simulink model "Simu2VITA"  (R2019b)
settings: Solver=VariableStepAuto  StartTime=0.0  StopTime=10.0  RelTol=1e-3
values from neighbouring files (symbols this model uses):
  actuators_tconst = ones(qty_actuators, 1)*0.1754    [vehicle_parameters_vita1_simu2vita.m]
  Dlf = -[X_u;         Y_v;         Z_w;         K_p;         M_q;         N_r]    [vehicle_parameters_vita1_simu2vita.m]
  Dqf = -[X_u_u;         Y_v_v;         Z_w_w;         K_p_p;         M_q_q;         N_r_r]    [vehicle_parameters_vita1_simu2vita.m]
  I_b = diag([I_x; I_y; I_z])    [vehicle_parameters_vita1_simu2vita.m]
  init_vehicle_linear_vel = [0 0 0]'    [init_params.m]
  init_vehicle_position = [0 0 0]'    [init_params.m]
  m = 25    [vehicle_parameters_vita1_simu2vita.m]
  Ma = -diag([X_u_dot; Y_v_dot; Z_w_dot; K_p_dot; M_q_dot; N_r_dot])    [vehicle_parameters_vita1_simu2vita.m]
  qty_actuators = 8    [vehicle_parameters_vita1_simu2vita.m]
  r_b = [0; 0; -0.08]    [vehicle_parameters_vita1_simu2vita.m]
  r_g = [0; 0; 0.02]    [vehicle_parameters_vita1_simu2vita.m]
  rho = 1028    [vehicle_parameters_vita1_simu2vita.m]
  thrust_inferior = ones(qty_actuators, 1)*(-39.91)    [vehicle_parameters_vita1_simu2vita.m]
  thrust_sup = ones(qty_actuators, 1)*51.48    [vehicle_parameters_vita1_simu2vita.m]
  vol = 0.02432    [vehicle_parameters_vita1_simu2vita.m]
undefined symbols (not defined in the file or in its folder): thruster_allocation_matrix
libraries: sharedutil x3, aerolibutil x3
settings Model: Creator=spades  LastModifiedBy=spades

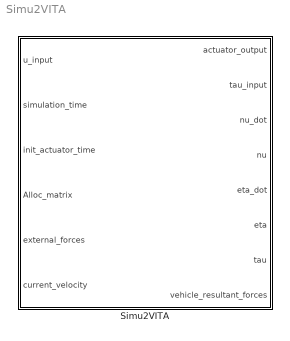
== system Simu2VITA ==
  Simu2VITA : Subsystem  mask{m_qty_actuators=qty_actuators, m_init_actuators_state=0, m_logic_op_use_custom_actuators_init_states=off, m_internal_init_actuators_time=0, m_logic_op_use_external_actuators_init_time=off, m_logic_op_use_external_time=off, m_thrust_sup=thrust_sup, m_thrust_inf=thrust_inferior, m_logic_op_thrust_saturation=on, m_actuators_tconst_vec=actuators_tconst, m_allocation_matrix=thruster_allocation_matrix, m_logic_op_external_alloc_mat=off, m_m=m, m_vol=vol, m_r_g=r_g, m_I_b=I_b, m_loigc_op_use_external_forces=off, m_Ma=Ma, m_Dlf_vec=Dlf, m_Dqf_vec=Dqf, m_current_velocity=[0 0 0]', m_loigc_op_use_external_current_velocity=off, m_g=9.81, m_rho=rho, m_r_b=r_b, m_eta_0=[init_vehicle_position' init_vehicle_orientation']', m_nu_0=[init_vehicle_linear_vel' init_vehicle_angular_vel']'}
      mask prompts: m_qty_actuators "Number of actuators on vehicle"; m_init_actuators_state "Actuators initial state values"; m_logic_op_use_custom_actuators_init_states "use custom initial state for actuators to start"; m_internal_init_actuators_time "Actuators initial time values"; m_logic_op_use_external_actuators_init_time "use external initial time for actuators to start"; m_logic_op_use_external_time "use external clock reference"; m_thrust_sup "Thrust upper saturation limits"; m_thrust_inf "Thrust lower saturation limits"; m_logic_op_thrust_saturation "use thrust saturation"; m_actuators_tconst_vec "Time Constant values"; m_allocation_matrix "Allocation Matrix"; m_logic_op_external_alloc_mat "use external allocation matrix"; m_m "Vehicle Total Mass"; m_vol "Vehicle Total Volume"; m_r_g "Vehicle center of gravity w.r.t. vehicle control point"; m_I_b "Inertia Matrix"; m_loigc_op_use_external_forces "enable external forces and moments"; m_Ma "Addded Mass Matrix"; m_Dlf_vec "Drag Linear Factor"; m_Dqf_vec "Drag Non Linear Factor"; m_current_velocity "Fluid current velocity"; m_loigc_op_use_external_current_velocity "use external fluid current velocity"; m_g "Gravity Constant"; m_rho "Fluid Constant"; m_r_b "Vehicle center of bouyance w.r.t. vehicle body frame"; m_eta_0 "Initial pose of the vehicle -- [pos quat]'"; m_nu_0 "Initial velocity and gyros of the vehicle -- [u v w p q r]'"
      mask init:
      | assert((numel(m_qty_actuators) == 1 && m_qty_actuators >= 0), 'The number of actuators must be a non-negative   scalar.');
      | 
      | if(m_qty_actuators == 0)
      |    
      |     m_logic_op_external_alloc_mat = false;
      |     m_allocation_matrix = zeros(6,1);
      |     m_init_actuators_state = 0;
      |     m_internal_init_actuators_time = 0;
      |     m_actuators_tconst_vec = 1;
      |     m_thrust_sup = 0;
      |     m_thrust_inf = 0;
      |     m_logic_op_thrust_saturation = false;
      |     
      | else
      |     
      |     if(~m_logic_op_use_custom_actuators_init_states)
      |         m_init_actuators_state = zeros(m_qty_actuators,1);
      |     end
      |     
      |     if(~m_logic_op_use_external_actuators_init_time)
      |         
      |         if(m_internal_init_actuators_time == 0)
      |             m_internal_init_actuators_time = zeros(m_qty_actuators,1);
      |         end
      |         
      |     end
      |     
      |     if(m_logic_op_thrust_saturation)
      |         assert(isequal(size(m_thrust_sup), [m_qty_actuators 1]));
      |         assert(isequal(size(m_thrust_inf), [m_qty_actuators 1]));
      |     end
      |     
      |     assert(isequal(size(m_init_actuators_state), [m_qty_actuators 1]), ...
      |         'Initial actuator state vector must be a column vector and agree with the number of actuators specified.');
      |     
      |     assert(isequal(size(m_internal_init_actuators_time), [m_qty_actuators 1]), ...
      |         'Initial actuator time vector must be a column vector and agree with the number of actuators specified.');
      |     
      | end
      | 
      | if(~m_logic_op_external_alloc_mat)
      | 
      |     assert(isequal(size(m_allocation_matrix), [6 numel(m_init_actuators_state)]));
      | 
      | end
      | 
      | assert(isequal(size(m_r_g), [3 1]), 'Center of gravity must be a 3x1 column vector.');
      | assert(isequal(size(m_r_b), [3 1]), 'Center of bouyancy must be a 3x1 column vector.');
      | assert(isequal(size(m_eta_0), [7 1]), 'Initial pose state w.r.t. NED must be a 7x1 column vector.');
      | assert(abs(norm(m_eta_0(4:7,1)) - 1) < 0.00001, 'Initial orientation state quaternion must have unitary norm.')
      | assert(isequal(size(m_nu_0), [6 1]), 'Initial velocity state w.r.t. body must be a 6x1 column vector.');
      | assert(isequal(size(m_I_b), [3 3]), 'Inertia matrix w.r.t. body must be a 3x3 matrix.');
      | assert(isequal(size(m_Ma), [6 6]), 'Added mass matrix must be a 6x6 matrix.');
      | assert(isequal(size(m_current_velocity), [3 1]), 'Current velocity must be a 3x1 column vector.');
      | assert(isequal(size(m_m), [1 1]), 'Mass must be a scalar.');
      | assert(isequal(size(m_vol), [1 1]), 'The volume of the vehicle must be a scalar.');
      | assert(isequal(size(m_g), [1 1]), 'Gravity must be a scalar.');
      | assert(isequal(size(m_rho), [1 1]), 'Fluid density must be a scalar.');
      | assert(isequal(size(m_Dlf_vec), [6 1]), 'Linear Drag Matrix is assumed to be diagonal and should be entered as a 6x1 vector.');
      | assert(isequal(size(m_Dqf_vec), [6 1]), 'Non-Linear Drag Matrix is assumed to be diagonal and should be entered as a 6x1 vector.');
      | 
      | m_W = m_m*m_g;
      | 
      | m_B = -m_vol*m_g*m_rho;
      | 
      | m_Smtrx_r_g = [0 -m_r_g(3) m_r_g(2); ... 
      |              m_r_g(3) 0 -m_r_g(1); ... 
      |             -m_r_g(2) m_r_g(1) 0];  
      | 
      | m_M = [m_m*eye(3) -m_m*m_Smtrx_r_g; ...
      |      m_m*m_Smtrx_r_g m_I_b];
      | 
      | m_Dlf = diag(m_Dlf_vec);
      | m_Dqf = diag(m_Dqf_vec);
      | 
      | m_Ad = diag((-1./m_actuators_tconst_vec))
      | m_Bd = -m_Ad
      | m_Cd = diag(ones(size(m_Ad, 2), 1))
      | m_Dd = zeros(numel(m_actuators_tconst_vec), numel(m_actuators_tconst_vec))
      mask Callback m_logic_op_use_custom_actuators_init_states:
      | p = Simulink.Mask.get(gcb);
      | a = p.Parameters(2);
      | 
      | cur_param_val_on = ...
      |     (strcmp(get_param(gcb, 'm_logic_op_use_custom_actuators_init_states'), 'on') ~= 0);
      | 
      | if (cur_param_val_on)
      | 
      |     for i = 1
      |         a(i).set('Enabled', 'on');
      |     end
      | 
      | else
      | 
      |     for i = 1
      |         a(i).set('Enabled', 'off');
      |     end
      | 
      | end
      mask Callback m_logic_op_use_external_actuators_init_time:
      | p = Simulink.Mask.get(gcb);
      | a = p.Parameters(4);
      | 
      | cur_param_val_on = ...
      |     (strcmp(get_param(gcb, 'm_logic_op_use_external_actuators_init_time'), 'on') ~= 0);
      | 
      | if (cur_param_val_on)
      | 
      |     for i = 1
      |         a(i).set('Enabled', 'off');
      |     end
      | 
      | else
      | 
      |     for i = 1
      |         a(i).set('Enabled', 'on');
      |     end
      | 
      | end
      mask Callback m_logic_op_thrust_saturation:
      | p = Simulink.Mask.get(gcb);
      | a = p.Parameters(7:8);
      | 
      | cur_param_val_on = ...
      |     (strcmp(get_param(gcb, 'm_logic_op_thrust_saturation'), 'on') ~= 0);
      | 
      | if (cur_param_val_on)
      | 
      |     for i = 1:2
      |         a(i).set('Enabled', 'on');
      |     end
      | 
      | else
      | 
      |     for i = 1:2
      |         a(i).set('Enabled', 'off');
      |     end
      | 
      | end
      mask Callback m_logic_op_external_alloc_mat:
      | p = Simulink.Mask.get(gcb);
      | a = p.Parameters(11);
      | 
      | cur_param_val_on = ...
      |     (strcmp(get_param(gcb, 'm_logic_op_external_alloc_mat'), 'on') ~= 0);
      | 
      | if (cur_param_val_on)
      | 
      |     for i = 1
      |         a(i).set('Enabled', 'off');
      |     end
      | 
      | else
      | 
      |     for i = 1
      |         a(i).set('Enabled', 'on');
      |     end
      | 
      | end
      mask Callback m_loigc_op_use_external_current_velocity:
      | p = Simulink.Mask.get(gcb);
      | a = p.Parameters(21);
      | 
      | cur_param_val_on = ...
      |     (strcmp(get_param(gcb, 'm_loigc_op_use_external_current_velocity'), 'on') ~= 0);
      | 
      | if (cur_param_val_on)
      | 
      |     for i = 1
      |         a(i).set('Enabled', 'off');
      |     end
      | 
      | else
      | 
      |     for i = 1
      |         a(i).set('Enabled', 'on');
      |     end
      | 
      | end
      mask DialogControl act_system Prompt: Actuator Module
      mask DialogControl act_start_group Prompt: Start options
      mask DialogControl thrust_sat_options Prompt: Thrust saturation options
      mask DialogControl act_evo_group Prompt: Evolution options
      mask DialogControl vehicle_input_tab Prompt: Allocation Module
      mask DialogControl vehicle_dynamic_tab Prompt: Vehicle Dynamic Parameters
      mask DialogControl rigid_body_comp Prompt: Rigid-body Components
      mask DialogControl m_vol Tooltip: Liters
      mask DialogControl hydro_dynam_comp Prompt: Hydrodanymic Components
      mask DialogControl hydro_static_comp Prompt: Hydrostatic Components
      mask DialogControl init_state Prompt: Initial state of the vehicle
      mask DialogControl m_eta_0 Tooltip: Pose state of the vehicle [pose quat]', with pose in meters w.r.t. NED

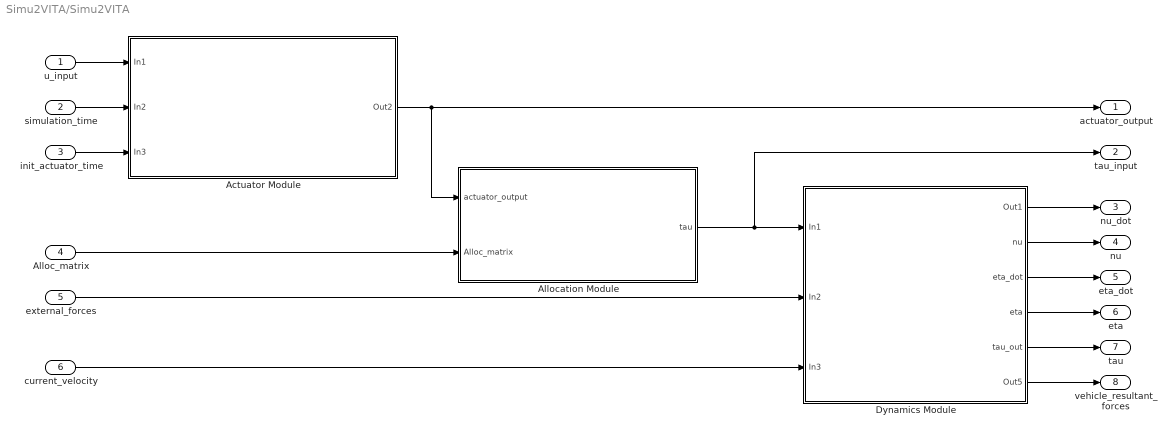
== system Simu2VITA/Simu2VITA ==
  u_input : Inport
  simulation_time : Inport  Port=2  PortDimensions=1
  init_actuator_time : Inport  Port=3
  Alloc_matrix : Inport  Port=4
  external_forces : Inport  Port=5
  current_velocity : Inport  Port=6
  Actuator Module : Subsystem
  Allocation Module : Subsystem
  Dynamics Module : Subsystem
  actuator_output : Outport  VectorParamsAs1DForOutWhenUnconnected=off
  "tau_input " : Outport  Port=2  VectorParamsAs1DForOutWhenUnconnected=off
  nu_dot : Outport  Port=3  VectorParamsAs1DForOutWhenUnconnected=off
  nu : Outport  Port=4  VectorParamsAs1DForOutWhenUnconnected=off
  eta_dot : Outport  Port=5  VectorParamsAs1DForOutWhenUnconnected=off
  eta : Outport  Port=6  VectorParamsAs1DForOutWhenUnconnected=off
  tau : Outport  Port=7  VectorParamsAs1DForOutWhenUnconnected=off
  vehicle_resultant_forces : Outport  Port=8
  wires:
  Actuator Module/1(Out2) -> Allocation Module/1(actuator_output), actuator_output/1
  u_input/1 -> Actuator Module/1(In1)
  simulation_time/1 -> Actuator Module/2(In2)
  init_actuator_time/1 -> Actuator Module/3(In3)
  Allocation Module/1(tau) -> "tau_input "/1, Dynamics Module/1(In1)
  Alloc_matrix/1 -> Allocation Module/2(Alloc_matrix)
  external_forces/1 -> Dynamics Module/2(In2)
  current_velocity/1 -> Dynamics Module/3(In3)
  Dynamics Module/1(Out1) -> nu_dot/1
  Dynamics Module/2(nu) -> nu/1
  Dynamics Module/3(eta_dot) -> eta_dot/1
  Dynamics Module/4(eta) -> eta/1
  Dynamics Module/6(Out5) -> vehicle_resultant_forces/1
  Dynamics Module/5(tau_out) -> tau/1

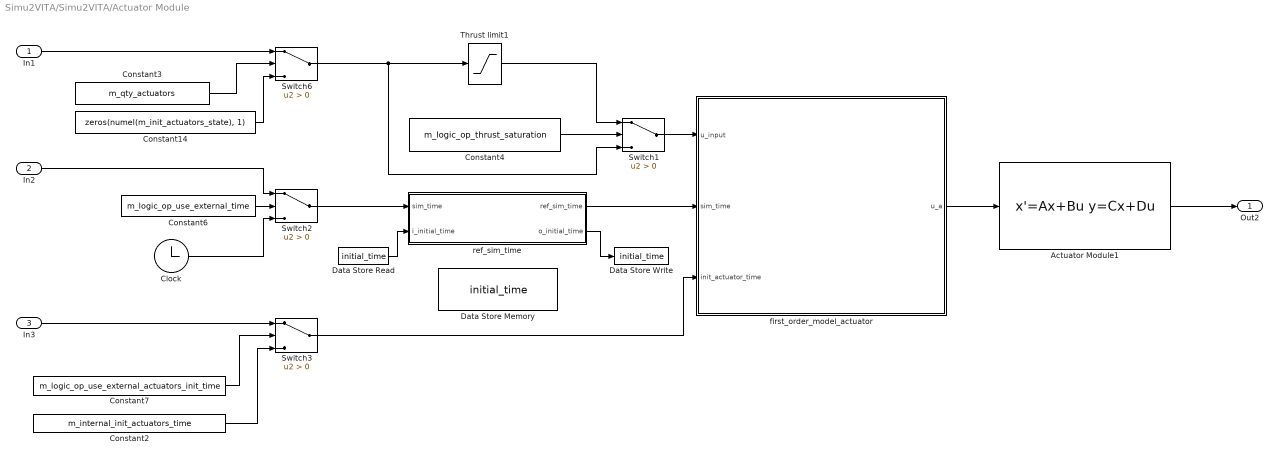
== system Simu2VITA/Simu2VITA/Actuator Module ==
  In1 : Inport
  In2 : Inport  Port=2
  In3 : Inport  Port=3
  Actuator Module1 : StateSpace  A=m_Ad  B=m_Bd  C=m_Cd  D=m_Dd  InitialCondition=m_init_actuators_state  ContinuousStateAttributes='actuator_state'
  Clock : Clock
  Constant14 : Constant  Value=zeros(numel(m_init_actuators_state), 1)
  Constant2 : Constant  Value=m_internal_init_actuators_time
  Constant3 : Constant  Value=m_qty_actuators
  Constant4 : Constant  Value=m_logic_op_thrust_saturation
  Constant6 : Constant  Value=m_logic_op_use_external_time
  Constant7 : Constant  Value=m_logic_op_use_external_actuators_init_time
  Data Store Memory : DataStoreMemory  DataStoreName=initial_time  ReadBeforeWriteMsg=warning  WriteAfterWriteMsg=warning  WriteAfterReadMsg=warning  InitialValue=-1  ShowAdditionalParam=off
  Data Store Read : DataStoreRead  DataStoreName=initial_time
  Data Store Write : DataStoreWrite  DataStoreName=initial_time
  Switch{1..3,6} (4 alike) : Switch  Criteria=u2 > Threshold
  Thrust limit1 : Saturate  UpperLimit=m_thrust_sup  LowerLimit=m_thrust_inf
  first_order_model_actuator : MATLAB Function  TreatAsAtomicUnit=on
  ref_sim_time : MATLAB Function  TreatAsAtomicUnit=on
  Out2 : Outport
  wires:
  Clock/1 -> Switch2/3
  Constant14/1 -> Switch6/3
  ref_sim_time/2(o_initial_time) -> Data Store Write/1
  Data Store Read/1 -> ref_sim_time/2(i_initial_time)
  Switch6/1 -> Switch1/3, Thrust limit1/1
  In1/1 -> Switch6/1
  Constant2/1 -> Switch3/3
  In2/1 -> Switch2/1
  Actuator Module1/1 -> Out2/1
  Switch2/1 -> ref_sim_time/1(sim_time)
  first_order_model_actuator/1(u_a) -> Actuator Module1/1
  Constant7/1 -> Switch3/2
  Constant3/1 -> Switch6/2
  In3/1 -> Switch3/1
  Constant6/1 -> Switch2/2
  Switch3/1 -> first_order_model_actuator/3(init_actuator_time)
  ref_sim_time/1(ref_sim_time) -> first_order_model_actuator/2(sim_time)
  Constant4/1 -> Switch1/2
  Thrust limit1/1 -> Switch1/1
  Switch1/1 -> first_order_model_actuator/1(u_input)

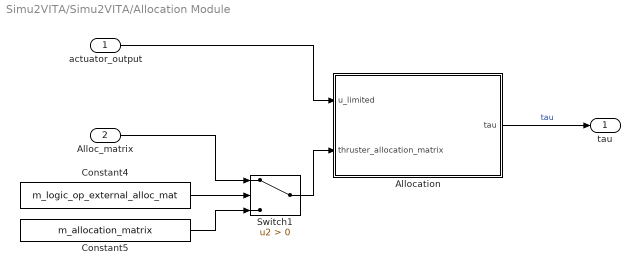
== system Simu2VITA/Simu2VITA/Allocation Module ==
  actuator_output : Inport
  Alloc_matrix : Inport  Port=2
  Allocation : MATLAB Function  TreatAsAtomicUnit=on
  Constant4 : Constant  Value=m_logic_op_external_alloc_mat
  Constant5 : Constant  Value=m_allocation_matrix
  Switch1 : Switch  Criteria=u2 > Threshold
  tau : Outport
  wires:
  Constant5/1 -> Switch1/3
  Constant4/1 -> Switch1/2
  Allocation/1(tau) -> tau/1  "tau"
  Switch1/1 -> Allocation/2(thruster_allocation_matrix)
  actuator_output/1 -> Allocation/1(u_limited)
  Alloc_matrix/1 -> Switch1/1

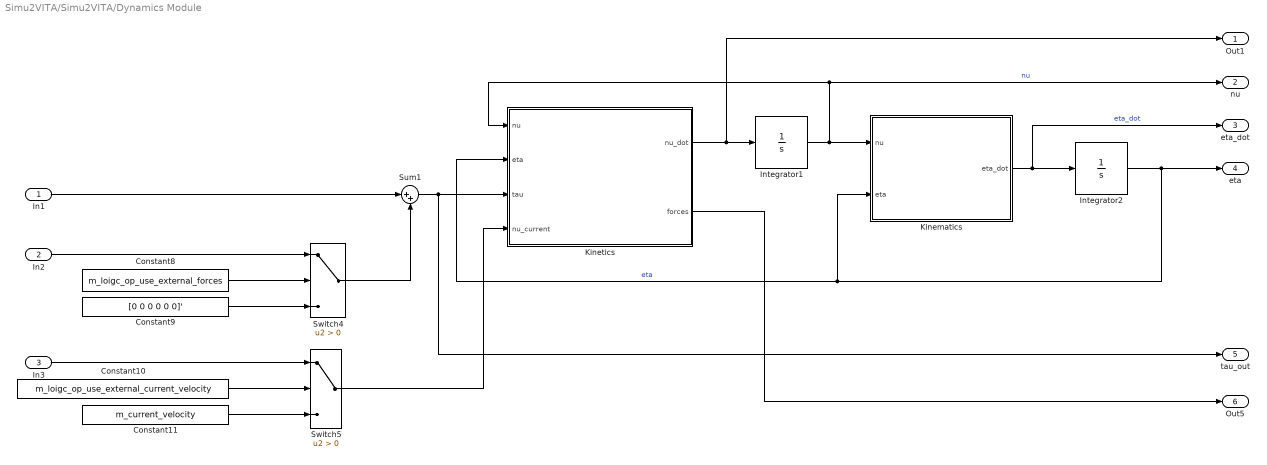
== system Simu2VITA/Simu2VITA/Dynamics Module ==
  In1 : Inport
  In2 : Inport  Port=2
  In3 : Inport  Port=3
  Constant10 : Constant  Value=m_loigc_op_use_external_current_velocity
  Constant11 : Constant  Value=m_current_velocity
  Constant8 : Constant  Value=m_loigc_op_use_external_forces
  Constant9 : Constant  Value=[0 0 0 0 0 0]'
  Integrator1 : Integrator  InitialCondition=m_nu_0
  Integrator2 : Integrator  InitialCondition=m_eta_0
  Kinematics : MATLAB Function  TreatAsAtomicUnit=on
  Kinetics : Subsystem
  Sum1 : Sum  Inputs=|++
  Switch4 : Switch  Criteria=u2 > Threshold
  Switch5 : Switch  Criteria=u2 > Threshold
  Out1 : Outport
  nu : Outport  Port=2
  eta_dot : Outport  Port=3
  eta : Outport  Port=4
  tau_out : Outport  Port=5
  Out5 : Outport  Port=6
  wires:
  Kinetics/2(forces) -> Out5/1
  In1/1 -> Sum1/1
  Constant10/1 -> Switch5/2
  Constant11/1 -> Switch5/3
  In2/1 -> Switch4/1
  Kinetics/1(nu_dot) -> Out1/1, Integrator1/1
  Sum1/1 -> tau_out/1, Kinetics/3(tau)
  In3/1 -> Switch5/1
  Integrator1/1 -> Kinematics/1(nu), Kinetics/1(nu), nu/1  "nu"
  Switch5/1 -> Kinetics/4(nu_current)
  Kinematics/1(eta_dot) -> eta_dot/1, Integrator2/1  "eta_dot"
  Constant8/1 -> Switch4/2
  Integrator2/1 -> Kinetics/2(eta), Kinematics/2(eta), eta/1  "eta"
  Switch4/1 -> Sum1/2
  Constant9/1 -> Switch4/3

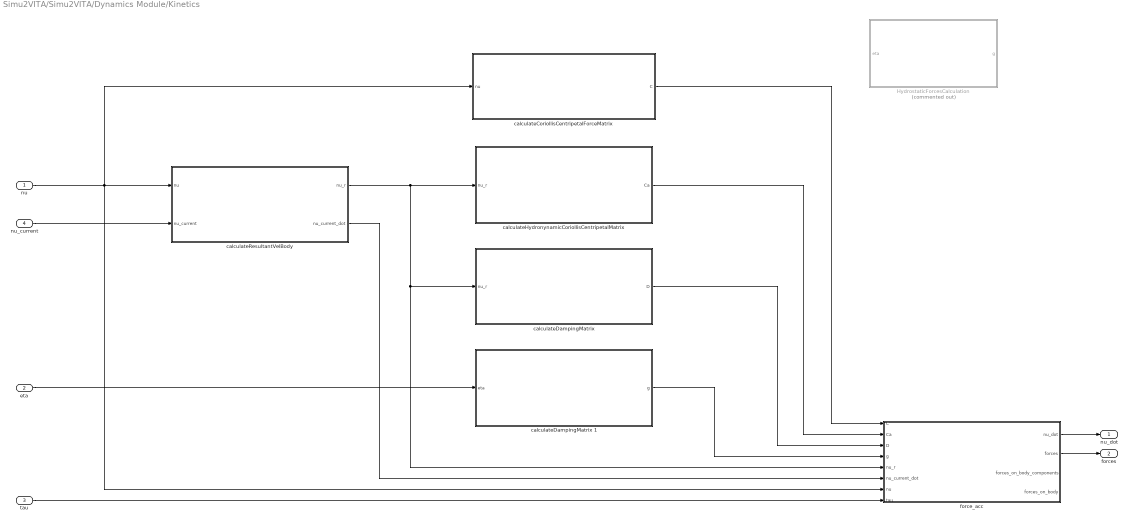
== system Simu2VITA/Simu2VITA/Dynamics Module/Kinetics ==
  nu : Inport
  eta : Inport  Port=2
  tau : Inport  Port=3
  nu_current : Inport  Port=4
  HydrostaticForcesCalculation : Subsystem  Commented=on
  calculateCoriollisCentripetalForceMatrix : MATLAB Function  TreatAsAtomicUnit=on
  "calculateDampingMatrix " : MATLAB Function  TreatAsAtomicUnit=on
  calculateDampingMatrix 1 : MATLAB Function  TreatAsAtomicUnit=on
  calculateHydronynamicCoriollisCentripetalMatrix : MATLAB Function  TreatAsAtomicUnit=on
  calculateResultantVelBody : MATLAB Function  TreatAsAtomicUnit=on
  force_acc : MATLAB Function  TreatAsAtomicUnit=on
  nu_dot : Outport
  forces : Outport  Port=2
  wires:
  calculateCoriollisCentripetalForceMatrix/1(C) -> force_acc/1(C)
  nu/1 -> force_acc/7(nu), calculateCoriollisCentripetalForceMatrix/1(nu), calculateResultantVelBody/1(nu)
  calculateResultantVelBody/1(nu_r) -> force_acc/5(nu_r), "calculateDampingMatrix "/1(nu_r), calculateHydronynamicCoriollisCentripetalMatrix/1(nu_r)
  force_acc/2(forces) -> forces/1
  force_acc/1(nu_dot) -> nu_dot/1
  nu_current/1 -> calculateResultantVelBody/2(nu_current)
  calculateResultantVelBody/2(nu_current_dot) -> force_acc/6(nu_current_dot)
  tau/1 -> force_acc/8(tau)
  calculateHydronynamicCoriollisCentripetalMatrix/1(Ca) -> force_acc/2(Ca)
  "calculateDampingMatrix "/1(D) -> force_acc/3(D)
  eta/1 -> calculateDampingMatrix 1/1(eta)
  calculateDampingMatrix 1/1(g) -> force_acc/4(g)

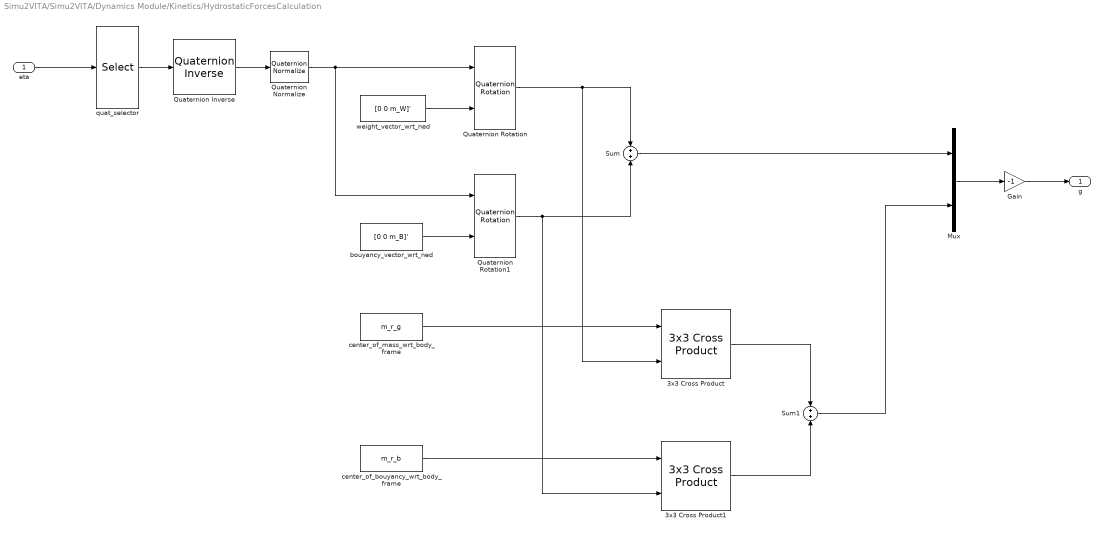
== system Simu2VITA/Simu2VITA/Dynamics Module/Kinetics/HydrostaticForcesCalculation ==
  eta : Inport
  3x3 Cross Product : sharedutil/3x3 Cross Product  aMode=aMode
      settings: SourceProductBaseCode=AE
  3x3 Cross Product1 : sharedutil/3x3 Cross Product  aMode=aMode
      settings: SourceProductBaseCode=AE
  Gain : Gain  Gain=-1
  Mux : Mux  Inputs=2
  Quaternion Inverse : aerolibutil/Quaternion Inverse
      settings: SourceProductName=Aerospace Blockset
  Quaternion Normalize : sharedutil/Quaternion Normalize  aMode=aMode
      settings: SourceProductName=Aerospace Blockset  SourceProductBaseCode=AE
  Quaternion Rotation : aerolibutil/Quaternion Rotation
  Quaternion Rotation1 : aerolibutil/Quaternion Rotation
  Sum : Sum  Inputs=+|+
  Sum1 : Sum  Inputs=+|+
  bouyancy_vector_wrt_ned : Constant  Value=[0 0 m_B]'
  center_of_bouyancy_wrt_body_frame : Constant  Value=m_r_b
  center_of_mass_wrt_body_frame : Constant  Value=m_r_g
  quat_selector : Selector  InputPortWidth=7  IndexOptions=Index vector (dialog)  Indices=[4 5 6 7]  OutputSizes=1
  weight_vector_wrt_ned : Constant  Value=[0 0 m_W]'
  g : Outport
  wires:
  eta/1 -> quat_selector/1
  quat_selector/1 -> Quaternion Inverse/1
  weight_vector_wrt_ned/1 -> Quaternion Rotation/2
  bouyancy_vector_wrt_ned/1 -> Quaternion Rotation1/2
  Quaternion Rotation/1 -> 3x3 Cross Product/2, Sum/1
  Sum/1 -> Mux/1
  Mux/1 -> Gain/1
  Quaternion Rotation1/1 -> 3x3 Cross Product1/2, Sum/2
  center_of_mass_wrt_body_frame/1 -> 3x3 Cross Product/1
  center_of_bouyancy_wrt_body_frame/1 -> 3x3 Cross Product1/1
  3x3 Cross Product/1 -> Sum1/1
  3x3 Cross Product1/1 -> Sum1/2
  Sum1/1 -> Mux/2
  Gain/1 -> g/1
  Quaternion Inverse/1 -> Quaternion Normalize/1
  Quaternion Normalize/1 -> Quaternion Rotation1/1, Quaternion Rotation/1

== matlab function Simu2VITA/Actuator Module/first_order_model_actuator ==
  data: u_a output; u_input input; sim_time input; init_actuator_time input
function u_a  = channel_selector(u_input, sim_time, init_actuator_time)

        u_a = u_input.*(sim_time > init_actuator_time);
           
end

== matlab function Simu2VITA/Dynamics Module/Kinetics/calculateDampingMatrix 1 ==
  data: g output; eta input; m_W parameter; m_B parameter; m_r_g parameter; m_r_b parameter
function g = calculateHydrostaticForcesCalculation(eta, m_W, m_B, m_r_g, m_r_b)
            
   coder.extrinsic('MException')
    
    ori = eta(4:7);
    
    g = zeros(6,1);
    
    [Mori, Nori] = size(ori);
    
    if(Mori == 3 && Nori == 1)
        
    elseif(Mori == 4 && Nori == 1)

        q = [eta(4); -eta(5:end)]/norm(eta(4:end));

        S = [0 -q(4) q(3); ...
             q(4) 0 -q(2); ...
            -q(3) q(2) 0;];
        
        r = [0;0;m_W];
        weight_wrt_body = (q(1) - norm(q(2:4)))*r + 2*q(2:4)*(q(2:4)'*r) + 2*q(1)*S*r;
        
        r = [0;0;m_B];
        bouyancy_wrt_body = (q(1) - norm(q(2:4)))*r + 2*q(2:4)*(q(2:4)'*r) + 2*q(1)*S*r;
        
        g(1:3) = -(weight_wrt_body + bouyancy_wrt_body);
        g(4:6) = -(cross(m_r_g, weight_wrt_body) + cross(m_r_b, bouyancy_wrt_body));
        

    end

end

== matlab function Simu2VITA/Dynamics Module/Kinematics ==
  data: nu input; eta_dot output; eta input
function eta_dot = vita_robot_kinematics(nu, eta)

    R_b2n = [1-2*(eta(6)^2 + eta(7)^2) 2*(eta(5)*eta(6)-eta(7)*eta(4)) 2*(eta(5)*eta(7)+eta(6)*eta(4)); ...
             2*(eta(5)*eta(6)+eta(7)*eta(4)) 1-2*(eta(5)^2 + eta(7)^2) 2*(eta(6)*eta(7)-eta(5)*eta(4)); ...
             2*(eta(5)*eta(7)-eta(6)*eta(4)) 2*(eta(6)*eta(7)+eta(5)*eta(4)) 1-2*(eta(5)^2 + eta(6)^2)];
         
    T = 0.5*[-eta(5) -eta(6) -eta(7); ... 
              eta(4) -eta(7)  eta(6); ...
              eta(7)  eta(4) -eta(5); ...
             -eta(6)  eta(5)  eta(4);];
      
   q = eta(4:7);
   
   eta_dot = zeros(7,1);
   
   %rate of convergence of the quaternion (Chapter 3 of Fossen 2011)
   gamma = 100;
   
   eta_dot(1:3) = R_b2n*nu(1:3);
   eta_dot(4:7) = T*nu(4:6) + (gamma/2)*(1-q'*q)*q;

end

== matlab function Simu2VITA/Dynamics Module/Kinetics/calculateCoriollisCentripetalForceMatrix ==
  data: nu input; C output; m_m parameter; m_r_g parameter; m_I_b parameter
function C = calculateCoriollisCentripetalForceMatrix(nu, m_m, m_r_g, m_I_b)
            
            v2 = nu(4:6);            
            
            Smtrx_v2 = [0 -v2(3) v2(2); ... 
                       v2(3) 0 -v2(1); ... 
                       -v2(2) v2(1) 0];
            
            I_bv2 = m_I_b*v2;
                  
            Smtrx_I_bv2 = [0 -I_bv2(3) I_bv2(2); ... 
                           I_bv2(3) 0 -I_bv2(1); ... 
                          -I_bv2(2) I_bv2(1) 0];
            
            Smtrx_r_g = [0 -m_r_g(3) m_r_g(2); ... 
                         m_r_g(3) 0 -m_r_g(1); ... 
                         -m_r_g(2) m_r_g(1) 0];
                   
            C11 = m_m*Smtrx_v2;
            C12 = -m_m*Smtrx_v2*Smtrx_r_g;
            C21 = m_m*Smtrx_r_g*Smtrx_v2;
            C22 = -Smtrx_I_bv2;
            
            C = [C11 C12; ...
                 C21 C22];
            
end

== matlab function Simu2VITA/Dynamics Module/Kinetics/calculateDampingMatrix  ==
  data: D output; nu_r input; m_Dlf parameter; m_Dqf parameter
function D = calculateDampingMatrix(nu_r, m_Dlf, m_Dqf)
            
    [velRow, velCols] = size(nu_r);

    if(velRow == 1 || velCols ~= 1)
        
        ME = MException('MyComponent:incompatiblePosition', ...
                'Position vector does not match a column vector!');

        throw(ME);
        
    else

        tmpMtrx = abs([nu_r nu_r nu_r nu_r nu_r nu_r]);

        D = m_Dlf + m_Dqf.*tmpMtrx;

    end

end

== matlab function Simu2VITA/Dynamics Module/Kinetics/calculateHydronynamicCoriollisCentripetalMatrix ==
  data: Ca output; nu_r input; m_Ma parameter
function Ca = calculateHydronynamicCoriollisCentripetalMatrix(nu_r, m_Ma)

    [velRow, velCols] = size(nu_r);

    if(velRow == 1 || velCols ~= 1)

        ME = MException('MyComponent:incompatiblePosition', ...
                'Position vector does not match a column vector!');

        throw(ME);

    else

        v = m_Ma*nu_r;
        
        Smtrx_v1 = [0 -v(3) v(2); ... 
                    v(3) 0 -v(1); ... 
                    -v(2) v(1) 0];

        Smtrx_v2 = [0 -v(6) v(5); ... 
                    v(6) 0 -v(4); ... 
                    -v(5) v(4) 0];

        Ca = [zeros(3,3) -Smtrx_v1; ...
              -Smtrx_v1  -Smtrx_v2]; 


    end

end

== matlab function Simu2VITA/Dynamics Module/Kinetics/calculateResultantVelBody ==
  data: nu input; nu_r output; nu_current_dot output; nu_current input
function [nu_r, nu_current_dot] = calculateResultantVelBody(nu, nu_current)
    
   nu_r = nu - [nu_current' 0 0 0]';

   nu_current_dot = [[[0 -nu(6) nu(5); ... 
                       nu(6) 0 -nu(3); ...
                       -nu(5) nu(3) 0]*nu_current]' 0 0 0]';
   
   

end

== matlab function Simu2VITA/Dynamics Module/Kinetics/force_acc ==
  data: C input; Ca input; D input; g input; m_Ma parameter; nu_r input; nu_current_dot input; nu_dot output; nu input; forces output; forces_on_body_components output; tau input; m_M parameter; forces_on_body output
function [nu_dot, forces, forces_on_body_components, forces_on_body] = force_acc(C, Ca, D, g, m_Ma, nu_r, nu_current_dot, nu, tau, m_M)
    
    forces_on_body_components = [m_Ma*nu_current_dot; ...
                                   C*nu; ...
                                 Ca*nu_r; ...
                                 D*nu_r; ...
                                 g];
    forces_on_body = m_Ma*nu_current_dot - C*nu - Ca*nu_r - D*nu_r -  g;
    forces = (tau + forces_on_body);
    nu_dot = (m_M + m_Ma)\forces;
    
end

== matlab function Simu2VITA/Actuator Module/ref_sim_time ==
  data: sim_time input; ref_sim_time output; i_initial_time input; o_initial_time output
function [ref_sim_time, o_initial_time] = ref_sim_time(sim_time, i_initial_time)

        if(i_initial_time == -1)
            i_initial_time = sim_time;
        end

        ref_sim_time = sim_time - i_initial_time;
        o_initial_time =  i_initial_time;
           
end

== matlab function Simu2VITA/Allocation Module/Allocation ==
  data: u_limited input; tau output; thruster_allocation_matrix input
function tau = vehicle_allocation_function(u_limited, thruster_allocation_matrix)

 tau = thruster_allocation_matrix*u_limited;

end
